simulink model "otu19"  (R2018a)
settings: Solver=ode45  StartTime=0.0  StopTime=5  RelTol=1e-3  EnableMultiTasking=on
settings Model: Creator=bukova.2018  LastModifiedBy=chernakov.2018
settings DataIOCC: LimitDataPoints=on  SaveFormat=Array  SignalLoggingSaveFormat=ModelDataLogs
settings OptimizationCC: ExpressionDepthLimit=2147483647  LifeSpan=inf
settings DebuggingCC: UnderspecifiedInitializationDetection=Classic  MergeDetectMultiDrivingBlocksExec=none  SolverPrmCheckMsg=warning  FcnCallInpInsideContextMsg=warning  StateNameClashWarn=warning  SFUnexpectedBacktrackingDiag=warning  SFNoUnconditionalDefaultTransitionDiag=warning  SFExecutionAtInitializationDiag=none
settings HardwareCC: ProdBitPerPointer=32  ProdBitPerSizeT=32  ProdBitPerPtrDiffT=32  ProdLargestAtomicFloat=None  ProdIntDivRoundTo=Undefined  ProdEndianess=Unspecified  ProdWordSize=32  ProdHWDeviceType=32-bit Generic
settings ModelReferenceCC: PropagateSignalLabelsOutOfModel=off
settings CodeAppCC: StateflowObjectComments=on
settings GRTTargetCC: TargetLangStandard=C89/C90 (ANSI)  GeneratePreprocessorConditionals=Disable all  CombineOutputUpdateFcns=off  GRTInterface=on
settings ConfigComp: CovMetricSettings=dw  CovHtmlReporting=on  CovSaveCumulativeToWorkspaceVar=on  CovSaveSingleToWorkspaceVar=on  CovExternalEMLEnable=off

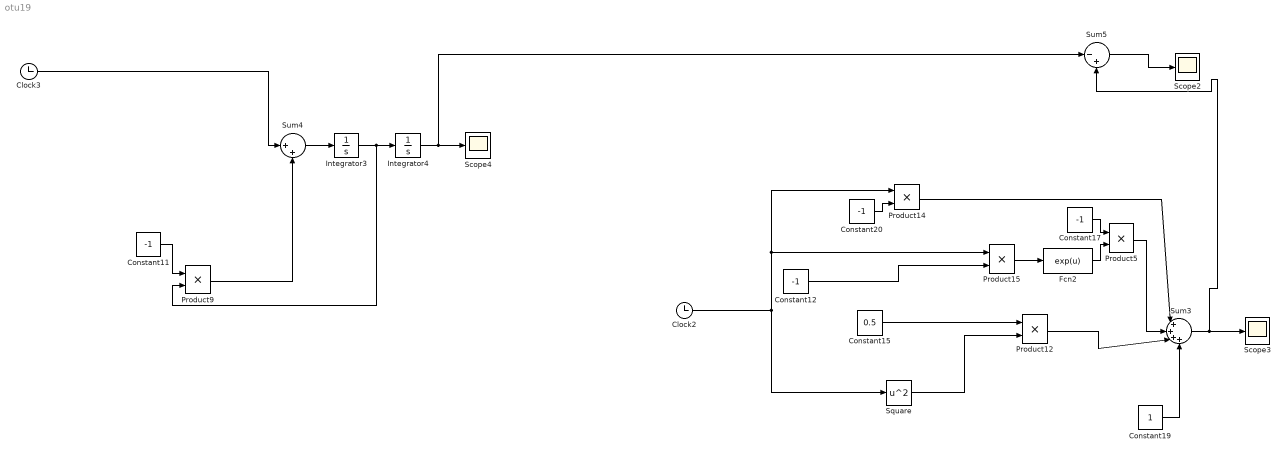
== system otu19 ==
  Clock2 : Clock
  Clock3 : Clock
  Constant{11..12,17,20} (4 alike) : Constant  Value=-1
  Constant15 : Constant  Value=0.5
  Constant19 : Constant
  Fcn2 : Fcn  Expr=exp(u)
  Integrator3 : Integrator
  Integrator4 : Integrator
  Product{5,9,12,14..15} (5 alike) : Product  RndMeth=Zero
  Scope2 : Scope
  Scope3 : Scope
  Scope4 : Scope
  Square : Math  Operator=square  SaturateOnIntegerOverflow=on
  Sum3 : Sum  Inputs=|++++
  Sum4 : Sum  Inputs=|++
  Sum5 : Sum  Inputs=|-+
  wires:
  Constant19/1 -> Sum3/4
  Product5/1 -> Sum3/2
  Clock2/1 -> Square/1, Product14/1, Product15/1
  Constant11/1 -> Product9/1
  Constant15/1 -> Product12/1
  Product14/1 -> Sum3/1
  Product12/1 -> Sum3/3
  Constant12/1 -> Product15/2
  Clock3/1 -> Sum4/1
  Integrator4/1 -> Sum5/1, Scope4/1
  Constant17/1 -> Product5/1
  Fcn2/1 -> Product5/2
  Product15/1 -> Fcn2/1
  Sum5/1 -> Scope2/1
  Constant20/1 -> Product14/2
  Sum4/1 -> Integrator3/1
  Integrator3/1 -> Product9/2, Integrator4/1
  Square/1 -> Product12/2
  Sum3/1 -> Sum5/2, Scope3/1
  Product9/1 -> Sum4/2
